simulink model "moror_lab5"  (R2024b)
settings: Solver=VariableStepAuto  StartTime=0.0  StopTime=10.0  RelTol=1e-3
settings Model: Creator=Admin  LastModifiedBy=pragy

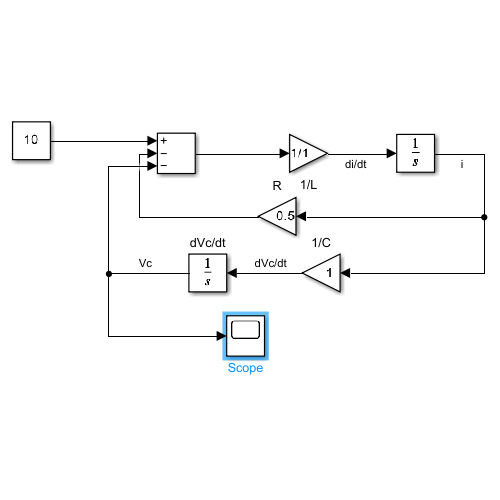
[thumbnail: Simulink's stored preview of the top-level diagram]
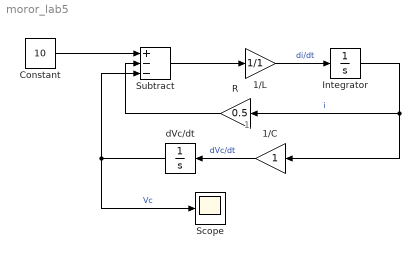
== system moror_lab5 ==
  note: 1
  1/C : Gain
  1/L : Gain  Gain=1/1
  Constant : Constant  Value=10
  Integrator : Integrator
  R : Gain  Gain=0.5
  Scope : Scope
  Subtract : Sum  Inputs=+--
  dVc/dt : Integrator
  wires:
  1/L/1 -> Integrator/1  "di/dt"
  Integrator/1 -> 1/C/1, R/1  "i"
  1/C/1 -> dVc/dt/1  "dVc/dt"
  Constant/1 -> Subtract/1
  R/1 -> Subtract/2
  dVc/dt/1 -> Scope/1, Subtract/3  "Vc"
  Subtract/1 -> 1/L/1
